simulink model "mod5"  (R2022a)
settings: Solver=VariableStepAuto  StartTime=0.0  StopTime=10.0  FixedStep=0.01  RelTol=1e-3
model workspace (MAT data in the model file):
  K = 2
settings Model: DataDictionary=data1.sldd  Creator=Administrator  LastModifiedBy=Administrator
settings DataIOCC: InspectSignalLogs=on

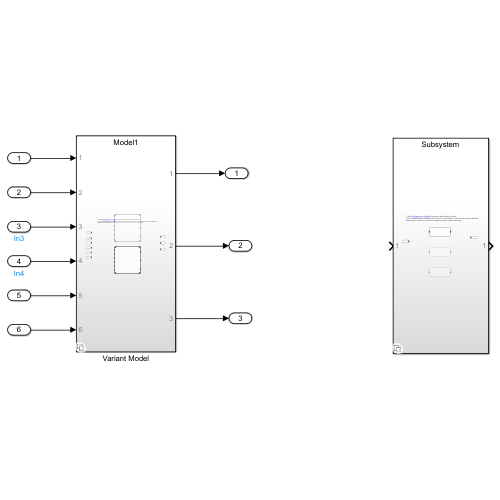
[thumbnail: Simulink's stored preview of the top-level diagram]
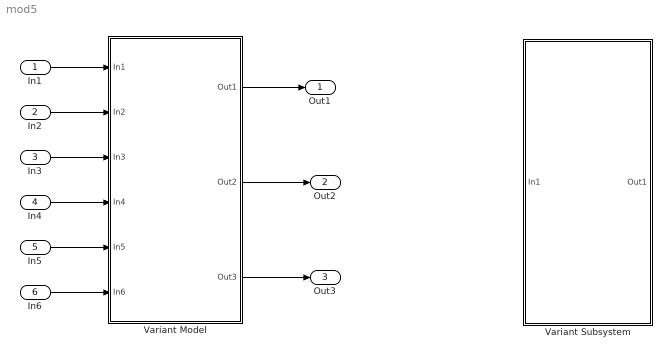
== system mod5 ==
  In1 : Inport
  In2 : Inport  Port=2
  In3 : Inport  Port=3
  In4 : Inport  Port=4
  In5 : Inport  Port=5
  In6 : Inport  Port=6
  Variant Model : Subsystem  Variant=on
  Variant Subsystem : Subsystem  Variant=on
  Out1 : Outport
  Out2 : Outport  Port=2
  Out3 : Outport  Port=3
  wires:
  In1/1 -> Variant Model/1(In1)
  In2/1 -> Variant Model/2(In2)
  In3/1 -> Variant Model/3(In3)
  In4/1 -> Variant Model/4(In4)
  In5/1 -> Variant Model/5(In5)
  In6/1 -> Variant Model/6(In6)
  Variant Model/1(Out1) -> Out1/1
  Variant Model/2(Out2) -> Out2/1
  Variant Model/3(Out3) -> Out3/1

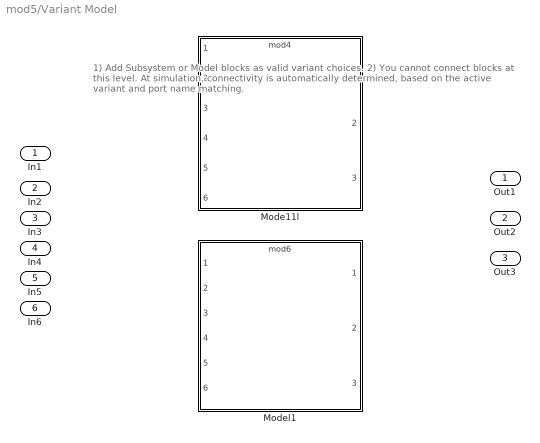
== system mod5/Variant Model ==
  note: 1) Add Subsystem or Model blocks as valid variant choices.
      | 2) You cannot connect blocks at this level. At simulation, connectivity is automatically
      | determined, based on the active variant and port name matching.
  In1 : Inport
  In2 : Inport  Port=2
  In3 : Inport  Port=3
  In4 : Inport  Port=4
  In5 : Inport  Port=5
  In6 : Inport  Port=6
  Mode11l : ModelReference  DisableCoverage=on  ModelNameDialog=mod4  VariantControl=K==1  ModelReferenceVersion=1.5
  Model1 : ModelReference  ModelNameDialog=mod6  VariantControl=K==2  ModelReferenceVersion=1.4
  Out1 : Outport
  Out2 : Outport  Port=2
  Out3 : Outport  Port=3

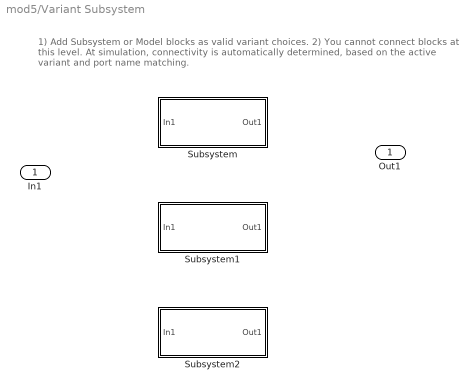
== system mod5/Variant Subsystem ==
  note: 1) Add Subsystem or Model blocks as valid variant choices.
      | 2) You cannot connect blocks at this level. At simulation, connectivity is automatically
      | determined, based on the active variant and port name matching.
  In1 : Inport
  Subsystem : Subsystem  VariantControl=true
  Subsystem1 : Subsystem  VariantControl=false
  Subsystem2 : Subsystem  VariantControl=false
  Out1 : Outport

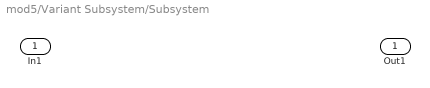
== system mod5/Variant Subsystem/Subsystem ==
  In1 : Inport
  Out1 : Outport

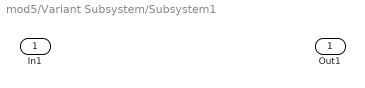
== system mod5/Variant Subsystem/Subsystem1 ==
  In1 : Inport
  Out1 : Outport

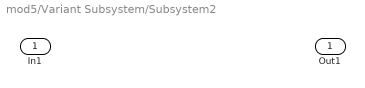
== system mod5/Variant Subsystem/Subsystem2 ==
  In1 : Inport
  Out1 : Outport
